simulink model "autonomousWaypointFollower"  (R2021b)
settings: Solver=VariableStepAuto  StartTime=0.0  StopTime=150  RelTol=1e-3
InitFcn:
  | FidelityStage = 2;
model workspace (MAT data in the model file):
  AirspeedVal = 58.2251893932
  LookaheadDc = 50
  LookaheadDistance = 500
  Waypoints = [-5313.43403732 -5313.49765579 -5315.24259606 -5316.98751886 -5318.73267892 -5320.47705726 -5322.22141779 -5323.96550555 -5324.69997396 -5326.29075872 -5327.88101514 -5329.47150848 ... (2598 elements, 866x3)]
  airspeedVal = 34.4977795798
  headingAngles = timeseries
  headingAngles.Name = 'unnamed'
  headingAngles.DataInfo = tsdata.datametadata
  headingAngles.DataInfo.Interpolation = tsdata.interpolation
  headingAngles.DataInfo.Interpolation.Fhandle : function handle (value not decoded)
  headingAngles.DataInfo.Interpolation.Name = 'linear'
  headingAngles.TimeInfo = tsdata.timemetadata
  headingAngles.TimeInfo.Length = 900
  headingAngles.TimeInfo.DuplicateTimes = 0
  headingAngles.TimeInfo.Time_ = [0.1 0.2 0.3 0.4 0.5 0.6 0.7 0.8 0.9 1 1.1 1.2 ... (900 elements, 900x1)]
  headingAngles.TimeInfo.Initialized = 1
  headingAngles.QualityInfo = tsdata.qualmetadata
  headingAngles.Data_ = [-0.669202399451 -0.666740658678 -0.663649347949 -0.65999326077 -0.655837190644 -0.651245931077 -0.646284275575 -0.641017017641 -0.635508950781 -0.629824868499 -0.62324164574 -0.615194362721 ... (900 elements, 900x1)]
  lookaheadPoint = timeseries
  lookaheadPoint.Name = 'unnamed'
  lookaheadPoint.DataInfo = tsdata.datametadata
  lookaheadPoint.DataInfo.Interpolation = tsdata.interpolation
  lookaheadPoint.DataInfo.Interpolation.Fhandle : function handle (value not decoded)
  lookaheadPoint.DataInfo.Interpolation.Name = 'linear'
  lookaheadPoint.TimeInfo = tsdata.timemetadata
  lookaheadPoint.TimeInfo.Length = 900
  lookaheadPoint.TimeInfo.DuplicateTimes = 0
  lookaheadPoint.TimeInfo.Time_ = [0.1 0.2 0.3 0.4 0.5 0.6 0.7 0.8 0.9 1 1.1 1.2 ... (900 elements, 900x1)]
  lookaheadPoint.TimeInfo.Initialized = 1
  lookaheadPoint.QualityInfo = tsdata.qualmetadata
  lookaheadPoint.Data_ = [-1648.86677503 -1646.13781659 -1643.39683878 -1640.64391692 -1637.87912629 -1635.10254219 -1632.31423992 -1629.51429479 -1626.70278208 -1623.8797771 -1621.04599578 -1618.20164622 ... (2700 elements, 900x3)]
  waypointData = [-1625.03275672 -1598.86938118 -1571.45340762 -1543.27035087 -1514.50729286 -1485.12594864 -1455.09042939 -1424.58849905 -1393.84251756 -1362.78862848 -1331.63098268 -1300.4045263 ... (291 elements, 97x3)]
undefined symbols (not defined in the file): aircraftTmax, ap, DiscIntNeverNeededParam, Earth, env, initialThrottle, midFidelityUAV, sensors, trimT, uavParam, WGS84
libraries: simulink x21, mbdriLib x20, aerolibconvert2 x2, aerolibtransform2 x1, uavalgslib x1
(part 1 of 3)
settings Model: DataDictionary=FideltypathFollowingData.sldd  ModifiedByFormat=The MathWorks, Inc.  PauseTimes=100  Creator=The MathWorks, Inc.  LastModifiedBy=The MathWorks, Inc.
settings DataIOCC: ReturnWorkspaceOutputs=off
settings OptimizationCC: UseDivisionForNetSlopeComputation=UseDivisionForReciprocalsOfIntegersOnly
settings DebuggingCC: AlgebraicLoopMsg=none  ParameterPrecisionLossMsg=none

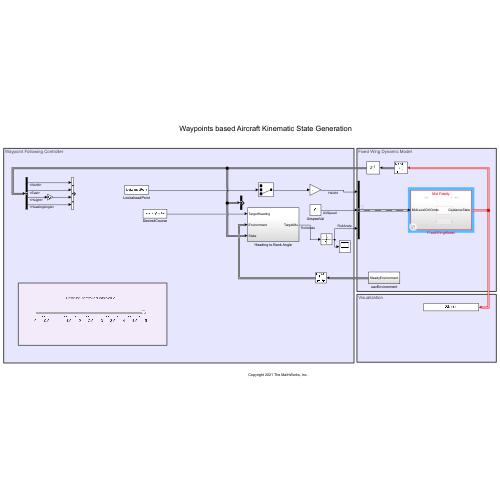
[thumbnail: Simulink's stored preview of the top-level diagram]
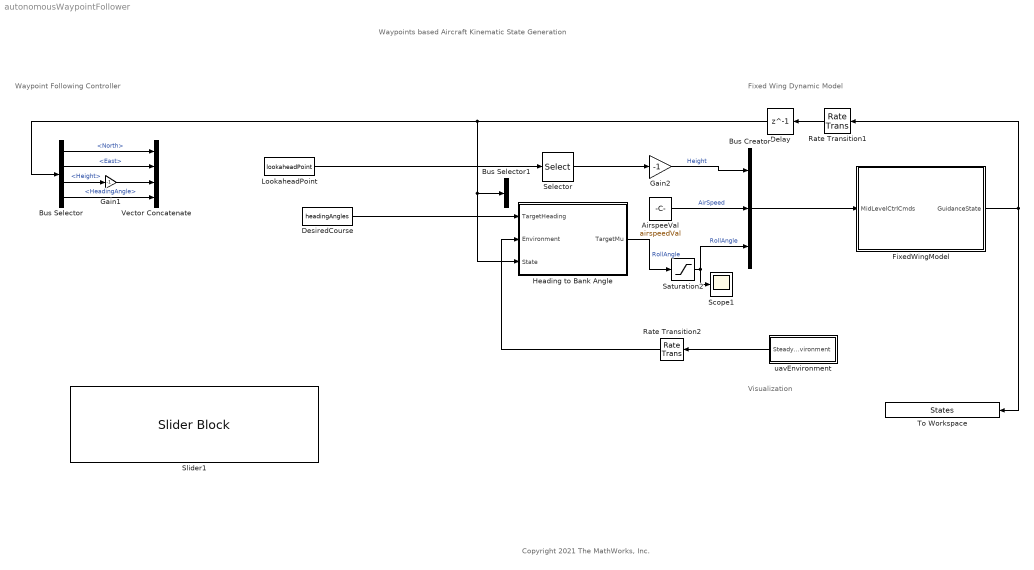
== system autonomousWaypointFollower ==
  note: Copyright 2021 The MathWorks, Inc.
  note: Waypoint Following Controller
  note: Waypoints based Aircraft Kinematic State Generation
  note: Fixed Wing Dynamic Model
  note: Visualization
  AirspeeVal : Constant  Value=airspeedVal  SampleTime=0.1
  Bus Creator : BusCreator  Inputs=3  OutDataTypeStr=Bus: FixedWingControlBus  NonVirtualBus=on
  Bus Selector : BusSelector  OutputSignals=North,East,Height,HeadingAngle
  Bus Selector1 : BusSelector  OutputSignals=AirSpeed
  Delay : Delay  DelayLength=1  InitialCondition=struct('North', midFidelityUAV.initialNorth, 'East', midFidelityUAV.initialEast,'Height', midFidelityUAV.initialAltitude, 'AirSpeed',midFidelityUAV.initialAirspeed,'HeadingAngle',midFidelityUAV.initialHeadingAngle,'FlightPathAngle', 0, 'RollAngle',0,'RollAngleRate',0)
  DesiredCourse : FromWorkspace  VariableName=headingAngles  OutDataTypeStr=double  SampleTime=0.1  OutputAfterFinalValue=Holding final value
  FixedWingModel : Subsystem  Variant=on
  Gain1 : Gain  Gain=-1
  Gain2 : Gain  Gain=-1
  Heading to Bank Angle : Subsystem
  LookaheadPoint : FromWorkspace  VariableName=lookaheadPoint  SampleTime=0.1  OutputAfterFinalValue=Holding final value
  Rate Transition1 : RateTransition  OutPortSampleTime=0.1
  Rate Transition2 : RateTransition  OutPortSampleTime=0.1
  Saturation2 : Saturate  UpperLimit=midFidelityUAV.maxroll/180*pi  LowerLimit=-midFidelityUAV.maxroll/180*pi
  Scope1 : Scope
  Selector : Selector  InputPortWidth=3  IndexOptions=Index vector (dialog)  Indices=[3]  OutputSizes=1
  Slider1 : SliderBlock  ScaleMax=5
  To Workspace : ToWorkspace  VariableName=States  SaveFormat=Timeseries  SampleTime=0.1
  Vector Concatenate : Concatenate  NumInputs=4
  uavEnvironment : Subsystem  VariantControl=NoWind
  wires:
  Rate Transition1/1 -> Delay/1
  Bus Selector/4 -> Vector Concatenate/4  "<HeadingAngle>"
  Bus Selector/2 -> Vector Concatenate/2  "<East>"
  Gain1/1 -> Vector Concatenate/3
  Delay/1 -> Bus Selector/1, Bus Selector1/1, Heading to Bank Angle/3(State)
  Selector/1 -> Gain2/1
  Bus Selector/1 -> Vector Concatenate/1  "<North>"
  Rate Transition2/1 -> Heading to Bank Angle/2(Environment)
  FixedWingModel/1(GuidanceState) -> Rate Transition1/1, To Workspace/1
  Bus Selector/3 -> Gain1/1  "<Height>"
  Heading to Bank Angle/1(TargetMu) -> Saturation2/1  "RollAngle"
  Saturation2/1 -> Bus Creator/3, Scope1/1  "RollAngle"
  Gain2/1 -> Bus Creator/1  "Height"
  uavEnvironment/1(SteadyEnvironment) -> Rate Transition2/1
  AirspeeVal/1 -> Bus Creator/2  "AirSpeed"
  DesiredCourse/1 -> Heading to Bank Angle/1(TargetHeading)
  LookaheadPoint/1 -> Selector/1
  Bus Creator/1 -> FixedWingModel/1(MidLevelCtrlCmds)

== system autonomousWaypointFollower/FixedWingModel ==
  MidLevelCtrlCmds : Inport
  High Fidelty : Subsystem  VariantControl=FidelityStage==3
  LowFidelity : Subsystem  VariantControl=FidelityStage==1
  Mid Fidelty : Subsystem  VariantControl=FidelityStage==2
  GuidanceState : Outport  VectorParamsAs1DForOutWhenUnconnected=off
